simulink model "maglev"  (R2024a)
settings: Solver=ode1  StartTime=0.0  StopTime=20  FixedStep=0.001  RelTol=1e-3
values from neighbouring files (symbols this model uses):
  A = [  0, 1,   0 ... (first row only)    [maglev_LTI.m]    (also in proyecto_maglev_rnn.m = [0, 1, 0; surfaces_smc.m = [0, 1, 0)
  B = [0 0 b3]'    [maglev_LTI.m]    (also in proyecto_maglev_rnn.m = [0; 0; 1/L]; surfaces_smc.m = [0; 0; 1/L])
  C = eye(size(A))    [maglev_LTI.m]    (also in proyecto_maglev_rnn.m = [1, 0, 0]; surfaces_smc.m = [1, 0, 0])
  D = zeros(size(C,1), size(B,2))    [maglev_LTI.m]    (also in proyecto_maglev_rnn.m; surfaces_smc.m)
  L = 0.4125    [proyecto_maglev_rnn.m]    (also in surfaces_smc.m = place(A', C', po)')
undefined symbols (not defined in the file or in its folder): Kueq, S
settings Model: Creator=jalej  LastModifiedBy=jalej

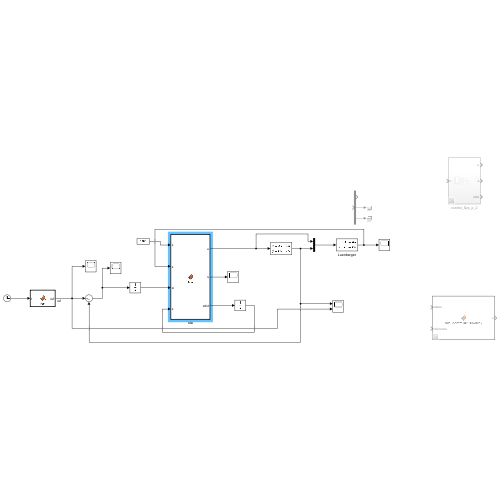
[thumbnail: Simulink's stored preview of the top-level diagram]
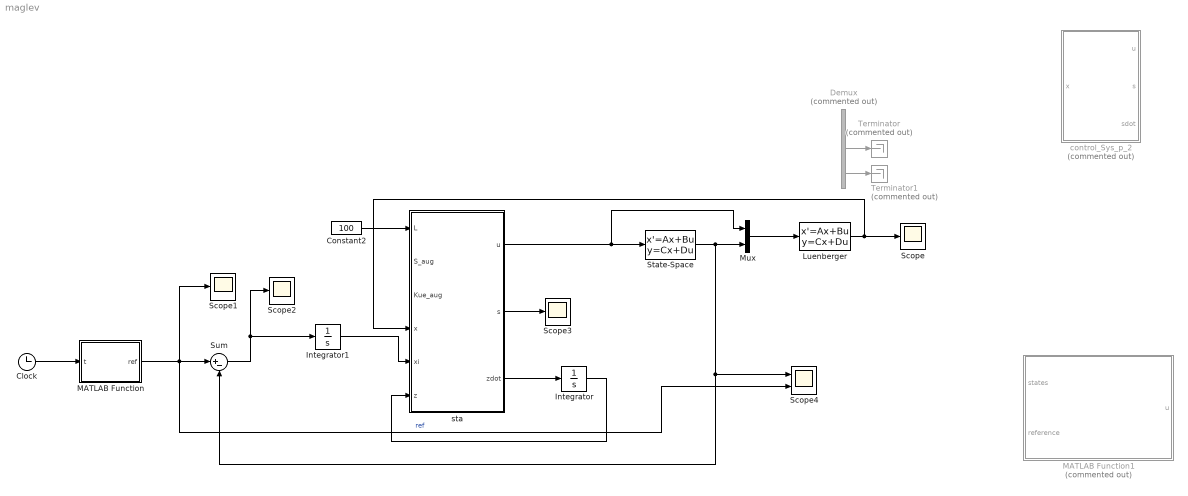
== system maglev ==
  Clock : Clock
  Constant2 : Constant  Value=100
  Demux : Demux  Commented=on  Outputs=3
  Integrator : Integrator
  Integrator1 : Integrator
  Luenberger : StateSpace  A=A-L*C  B=[B L]  C=eye(3)  D=zeros(3,2)  InitialCondition=[0, 0, 0]'
  MATLAB Function : MATLAB Function  TreatAsAtomicUnit=on
  MATLAB Function1 : MATLAB Function  Commented=on  TreatAsAtomicUnit=on
  Mux : Mux  Inputs=2
  Scope{,1..3} (4 alike) : Scope
  Scope4 : Scope  NumInputPorts=2
  State-Space : StateSpace  A=A  B=B  C=C  D=D  InitialCondition=[0, 0, 0]'
  Sum : Sum  Inputs=|+-
  Terminator : Terminator  Commented=on
  Terminator1 : Terminator  Commented=on
  control_Sys_p_2 : Subsystem  Commented=on
  sta : MATLAB Function  TreatAsAtomicUnit=on
  wires:
  Demux/2 -> Terminator/1
  Demux/3 -> Terminator1/1
  Clock/1 -> MATLAB Function/1(t)
  sta/1(u) -> Mux/1, State-Space/1
  sta/3(zdot) -> Integrator/1
  Integrator/1 -> sta/6(z)
  State-Space/1 -> Mux/2, Scope4/1, Sum/2
  Constant2/1 -> sta/1(L)
  MATLAB Function/1(ref) -> Scope1/1, Scope4/2, Sum/1  "ref"
  Sum/1 -> Scope2/1, Integrator1/1
  Integrator1/1 -> sta/5(xi)
  Mux/1 -> Luenberger/1
  Luenberger/1 -> sta/4(x), Scope/1
  sta/2(s) -> Scope3/1

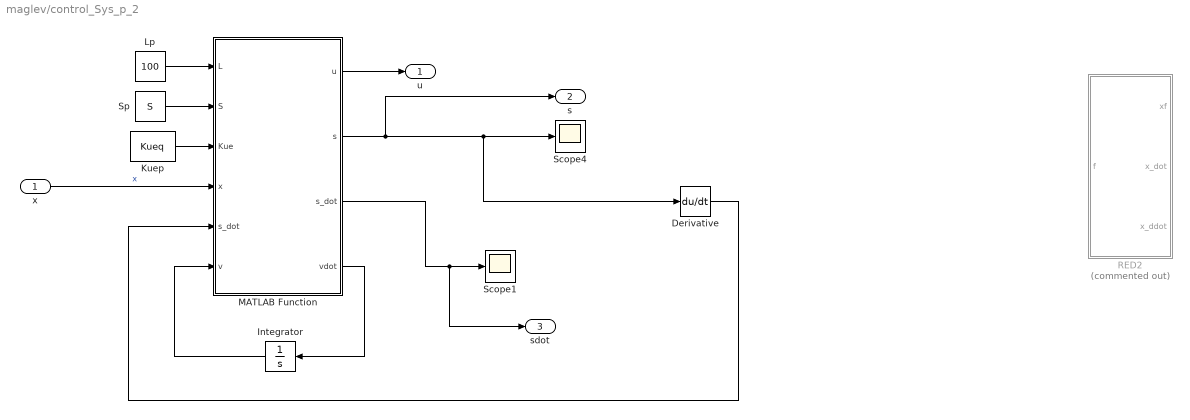
== system maglev/control_Sys_p_2 ==
  x : Inport
  Derivative : Derivative
  Integrator : Integrator
  Kuep : Constant  Value=Kueq  VectorParams1D=off
  Lp : Constant  Value=100  VectorParams1D=off
  MATLAB Function : MATLAB Function  TreatAsAtomicUnit=on
  RED2 : Subsystem  Commented=on
  Scope1 : Scope
  Scope4 : Scope
  Sp : Constant  Value=S  VectorParams1D=off
  u : Outport
  s : Outport  Port=2
  sdot : Outport  Port=3
  wires:
  Kuep/1 -> MATLAB Function/3(Kue)
  Integrator/1 -> MATLAB Function/6(v)
  MATLAB Function/4(vdot) -> Integrator/1
  Sp/1 -> MATLAB Function/2(S)
  MATLAB Function/1(u) -> u/1
  Lp/1 -> MATLAB Function/1(L)
  x/1 -> MATLAB Function/4(x)  "x"
  MATLAB Function/2(s) -> s/1, Derivative/1, Scope4/1
  MATLAB Function/3(s_dot) -> sdot/1, Scope1/1
  Derivative/1 -> MATLAB Function/5("s_dot ")

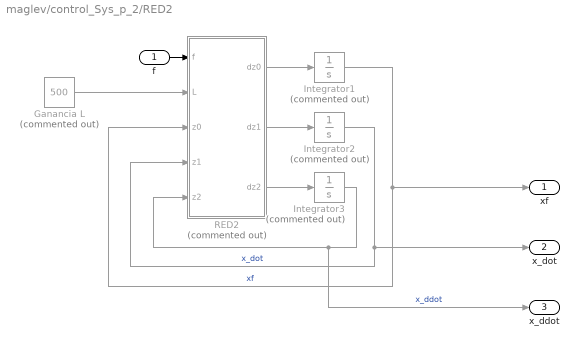
== system maglev/control_Sys_p_2/RED2 ==
  f : Inport
  Ganancia L : Constant  Commented=on  Value=500
  Integrator1 : Integrator  Commented=on
  Integrator2 : Integrator  Commented=on
  Integrator3 : Integrator  Commented=on
  RED2 : MATLAB Function  Commented=on  TreatAsAtomicUnit=on
  xf : Outport
  x_dot : Outport  Port=2
  x_ddot : Outport  Port=3
  wires:
  RED2/3(dz2) -> Integrator3/1
  Integrator1/1 -> xf/1, RED2/3(z0)  "xf"
  Integrator2/1 -> x_dot/1, RED2/4(z1)  "x_dot"
  Integrator3/1 -> x_ddot/1, RED2/5(z2)  "x_ddot"
  RED2/1(dz0) -> Integrator1/1
  RED2/2(dz1) -> Integrator2/1
  Ganancia L/1 -> RED2/2(L)
  f/1 -> RED2/1(f)

== matlab function maglev/MATLAB Function1 ==
  data: states input size=1; u output size=1; reference input size=1
function u = rnn_controller_simulink(states, reference)
%#codegen

% Variables persistentes para mantener Python inicializado
persistent python_initialized

% Inicializar Python engine una sola vez
if isempty(python_initialized)
    % Agregar ruta donde está el archivo Python
    pyrun("import sys");
    pyrun("sys.path.append(r'C:\Users\jalej\Documents\Documents-OneDrive\MAESTRIA\SEM_2\Inteligente\py')"); 
    % Inicializar controlador
    pyrun("from matlab_rnn_controller import init_rnn_controller, reset_rnn_controller");
    pyrun("init_rnn_controller()");
    pyrun("reset_rnn_controller()");
    
    python_initialized = true;
end

% Convertir entradas a Python
states_py = py.list(states);
reference_py = reference;

% Llamar función Python
u_py = pyrun("from matlab_rnn_controller import get_rnn_control; result = get_rnn_control(list(states_py), reference_py)", ...
             states_py=states_py, reference_py=reference_py);

% Convertir resultado a MATLAB
u = double(pyrun("result", result=u_py));

end

== matlab function maglev/MATLAB Function ==
  data: t input; ref output

function ref = fcn(t)
a0 = 0.007;  % Punto de equilibrio
if t < 3
    ref = 0.012 - a0;  % Desviación: +5mm
elseif t < 6
    ref = 0.009 - a0;  % Desviación: +2mm  
elseif t < 9
    ref = 0.002 - a0;  % Desviación: -5mm
else
    ref = 0;           % Equilibrio (desviación = 0)
end

== matlab function maglev/sta ==
  data: L input size=1; S_aug input; Kue_aug input; u output size=1; x input size=3; xi input size=1; z input size=1; s output size=1; zdot output size=1
function [u, s, zdot] = fcn(L, S_aug, Kue_aug, x, xi, z)
    % Estados aumentados: x (3x1) + xi (integral del error)
    x_aug = zeros(4,1);

    S_aug = [-285.64144     -5.0574812         0.4125      3569.9867];
    Kue_aug =[-10657.6854     -285.641438          60.125               0];

    x_aug = [x; xi];  % Estado aumentado 4x1
    
    % Superficie deslizante: s = S_x*x + S_xi*xi
    s = S_aug*x_aug;
    
    % Control equivalente para seguimiento
    ueqp = -Kue_aug*x_aug;
    
    % Super-twisting
    alpha = 1.5*sqrt(L);
    beta = 1.1 * L;

    u = -alpha * Csign(s, 1/2) + z + ueqp;
    zdot = -beta*sign(s);
end

== matlab function maglev/control_Sys_p_2/MATLAB Function ==
  data: L input; S input; Kue input; x input; s_dot input; u output; s output size=1; s_dot output size=1; v input; vdot output size=1
function [u, s, s_dot, vdot] = fcn(L, S, Kue, x, s_dot, v)
   
    ueq = -Kue*x;
    s = S*x;
    
    A = 1.0e+03 * [          0,    0.0010,         0;
                        1.4014,         0,    0.0139;
                             0,         0,   -0.0242];

    % % Calculemos x_dot analíticamente:
    x_dot = A*x;
    % 
    s_dot = S*x_dot;
    
    % Forzar que sean escalares
    s = s(1);
    s_dot = s_dot(1);
    
    alpha = 2.7 * L^(2/3);
    beta = 5.345 * L^(1/2);
    u = -alpha*Csign(s,1/3) - beta*Csign(s_dot, 1/2) + v + ueq;
    
    vdot = -1.1 * L * sign(s);
end

== matlab function maglev/control_Sys_p_2/RED2/RED2 ==
  data: f input; dz0 output; L input; z0 input; z1 input; z2 input; dz1 output; dz2 output
function [dz0,dz1,dz2] = fcn(f,L,z0,z1,z2)
% Derivador exacto de Levant para vector de n señales
% f: vector de entrada (nx1)
% L: parámetro de ganancia (escalar o vector nx1)
% z0,z1,z2: estados del derivador (nx1 cada uno)

k0 = 4.80;
k1 = 5.65;
k2 = 1.1;

% Obtener dimensión del vector
n = length(f);

% Inicializar salidas
dz0 = zeros(n,1);
dz1 = zeros(n,1);
dz2 = zeros(n,1);

% Permitir L escalar o vectorial
% if length(L) == 1
%     L_vec = L * ones(n,1);
% else
%     L_vec = L;
% end

% Aplicar derivador a cada señal
for i = 1:n
    e = z0(i) - f(i);
    dz0(i) = -k0 *L^(1/3) * Csign(e, 2/3) + z1(i);
    dz1(i) = -k1 *L^(2/3) * Csign(e, 1/3) + z2(i);
    dz2(i) = -k2 *L * Csign(e, 0);
end
end
